simulink model "MazeRobot_start"  (R2018a)
settings: Solver=ode23t  StartTime=0.0  StopTime=inf  RelTol=1e-3
InitFcn:
  | RPInit
model workspace (MAT data in the model file):
  mapForSim.obsMap = [0 0 0 0 0 0 0 0 0 0 0 0 ... (40000 elements, 200x200)]
  mapForSim.scaleFactor = 25
  mapForSim.simMap = robotics.BinaryOccupancyGrid
  mapForSim.simMap.Grid = [1 1 1 1 1 1 1 1 1 1 1 1 ... (40000 elements, 200x200)]
  mapForSim.simMap.GridSize = [200 200]
  mapForSim.simMap.Resolution = 25
  occGrid = robotics.BinaryOccupancyGrid
  occGrid.Grid = [1 1 1 1 1 1 1 1 1 1 1 1 ... (40000 elements, 200x200)]
  occGrid.GridSize = [200 200]
  occGrid.Resolution = 25
undefined symbols (not defined in the file): X, Y, Z
libraries: sm_lib x19, RP_Simulator_Components x15, nesl_utility x11, RoboticsPlayground x5, Contact_Forces_Lib x2
settings Model: EnablePacing=on  Creator=josea  LastModifiedBy=josea
settings DebuggingCC: UnconnectedLineMsg=none
settings DiagnosticsConfigSet: SimMechanicsRigidlyBoundBlock=none
settings ExplorerConfigSet: InternalSimMechanicsExplorerSettings="<ExplorerConfiguration><canonicalview>default</canonicalview><AnimationSetting><BasePlaybackSpeed>1.0</BasePlaybackSpeed><PlaybackSpeedFactor>1.0</PlaybackSpeedFactor></AnimationSetting><TilePanel><TileInfo><Tiles Columns=\"1\" Count=\"1\" Rows=\"1\"><Column Weight=\"1\"/><Row Weight=\"1\"/><Tile Height=\"1\" Width=\"1\" X=\"0\" Y=\"0\"/></Tiles></TileInfo><SceneInfo><SceneViewer><BGColor><R>0.60000002384185791</R><G>0.60000002384185791</G><B>0.60000002384185791</B></BGColor><Camera><DoPerspective>off</DoPerspective><Position><X>2.71941451456511407</X><Y>-6.77816927707449679</Y><Z>7.37038703658607108</Z></Position><Center><X>-0.142764420925711066</X><Y>0.264709257438438761</Y><Z>0.243094267201064668</Z></Center><Up><X>-0.202833782227054393</X><Y>0.654576301685044992</Y><Z>0.728277640779805169</Z></Up><ViewLimDist>1</ViewLimDist><YLim>4.3228780116357628</YLim><XLim>5.31983664569920922</XLim></Camera></SceneViewer></SceneInfo></TilePanel><MechEditorPanel><Cameras/><GfxPanelCameraMap/><VideoCreator><PlaybackSpeedRatio>4.0</PlaybackSpeedRatio><FrameRate>30</FrameRate><VideoFormat>Motion JPEG AVI</VideoFormat><FrameSize>[1280 720]</FrameSize></VideoCreator></MechEditorPanel></ExplorerConfiguration>"

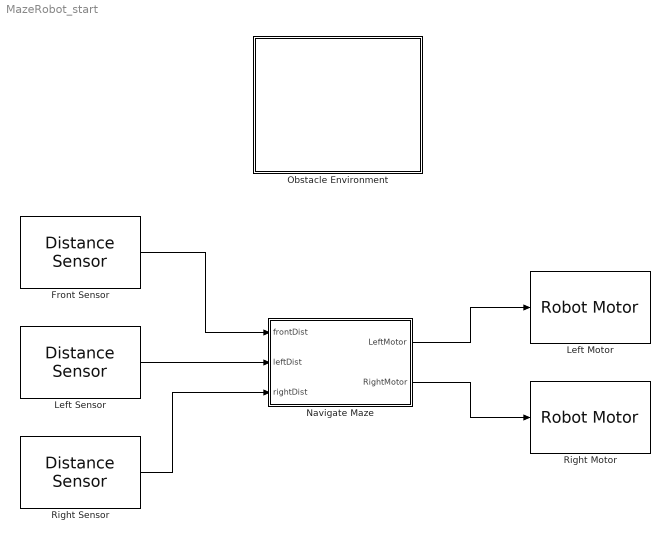
== system MazeRobot_start ==
  Front Sensor : RoboticsPlayground/Basic Sensors and Actuators/Distance Sensor  robotId=1  maxSenRange=10  minSenRange=0.02  senRes=0.01  sensOff=[0.25 0]  sensOffDeg=0  sensorTs=0.1
      settings: SourceProductName=Robotics Playground
  Left Motor : RoboticsPlayground/Basic Sensors and Actuators/Robot Motor  OverrideUsingVariant=Rbt1R  robotId=1  motorChoice=1
      settings: SourceProductName=Robotics Playground
  Left Sensor : RoboticsPlayground/Basic Sensors and Actuators/Distance Sensor  robotId=1  maxSenRange=10  minSenRange=0.02  senRes=0.01  sensOff=[0.15 0.15]  sensOffDeg=90  sensorTs=0.1
      settings: SourceProductName=Robotics Playground
  Navigate Maze : Stateflow chart  TreatAsAtomicUnit=on
  Obstacle Environment : Subsystem  mask(RP Obstacle Environment){obs1=on, obsPose1=[-2.042    0.091751], obsWidth1=3.713, obsLength1=0.91362, obs2=on, obsPose2=[0.025379    0.085895], obsWidth2=0.46852, obsLength2=4.6501, obs3=on, obsPose3=[1.3782      2.1357], obsWidth3=2.3075, obsLength3=0.57394, obs4=on, obsPose4=[1.2025     -1.9815], obsWidth4=2.776, obsLength4=0.51537, obs5=on, obsPose5=[2.8248   0.0097599], obsWidth5=2.1318, obsLength5=0.74963, obs6=on, obsPose6=[-2.1474      2.8736], obsWidth6=0.38653, obsLength6=1.9795, obs7=on, obsPose7=[-2.1415     -2.9244], obsWidth7=0.39824, obsLength7=1.9327, obs8=off, obsPose8=[2 2], obsWidth8=0.8, obsLength8=0.4, obs9=off, obsPose9=[2 2], obsWidth9=0.8, obsLength9=0.4, obs10=off, obsPose10=[2 2], obsWidth10=0.8, obsLength10=0.4, arenaLength=8, arenaWidth=8, robotId=1, wheelBase=0.5, wheelRadius=0.1, robotColor=[0 0 0.5], startPose=[-3.5 -3.5]}
      mask prompts: obs1 "Enable"; obsPose1 "Position X Y [m]"; obsWidth1 "Width [m]"; obsLength1 "Length [m]"; obs2 "Enable"; obsPose2 "Position X Y [m]"; obsWidth2 "Width [m]"; obsLength2 "Length [m]"; obs3 "Enable"; obsPose3 "Position X Y [m]"; obsWidth3 "Width [m]"; obsLength3 "Length [m]"; obs4 "Enable"; obsPose4 "Position X Y [m]"; obsWidth4 "Width [m]"; obsLength4 "Length [m]"; obs5 "Enable"; obsPose5 "Position X Y [m]"; obsWidth5 "Width [m]"; obsLength5 "Length [m]"; obs6 "Enable"; obsPose6 "Position X Y [m]"; obsWidth6 "Width [m]"; obsLength6 "Length [m]"; obs7 "Enable"; obsPose7 "Position X Y [m]"; obsWidth7 "Width [m]"; obsLength7 "Length [m]"; obs8 "Enable"; obsPose8 "Position X Y [m]"; obsWidth8 "Width [m]"; obsLength8 "Length [m]"; obs9 "Enable"; obsPose9 "Position X Y [m]"; obsWidth9 "Width [m]"; obsLength9 "Length [m]"; obs10 "Enable"; obsPose10 "Position X Y [m]"; obsWidth10 "Width [m]"; obsLength10 "Length [m]"; arenaLength "Length [m]"; arenaWidth "Width [m]"; robotId "Robot ID"; wheelBase "Distance between wheels [m]"; wheelRadius "Wheel radius [m]"; robotColor "Color [R G B]"; startPose "Initial Position X Y [m]"
      mask help:
      | This block contains a virtual environment for a single robot to interact with walls, obstacles and objects. Sensors implemented in the Robotics Playground library can be used to obtain environment information and actuators to interact with the robot behavior.
      |
      | Motor mapping for the robot is as follows:
      |
      | Motor 1 -> Left wheel motor torque
      | Motor 2 -> Right wheel motor torque
      settings: CopyFcn=|
      | set_param(gcs,'InitFcn','RPInit');
      | set_param(gcs,'Solver','ode23t');
      | set_param(gcs, 'EnablePacing', 'on')
      | set_param(gcs, 'PacingRate', 1)
      mask Help: web('obstacle_arena.htm')
      mask Callback obs1: commentObstacles(gcb)
      mask Callback obs2: commentObstacles(gcb)
      mask Callback obs3: commentObstacles(gcb)
      mask Callback obs4: commentObstacles(gcb)
      mask Callback obs5: commentObstacles(gcb)
      mask Callback obs6: commentObstacles(gcb)
      mask Callback obs7: commentObstacles(gcb)
      mask Callback obs8: commentObstacles(gcb)
      mask Callback obs9: commentObstacles(gcb)
      mask Callback obs10: commentObstacles(gcb)
      mask DialogControl obsT Prompt: Obstacle settings
      mask DialogControl Container19 Prompt: Set Obstacles Interactively
      mask DialogControl Control2 Prompt: Set Obstacles
      mask DialogControl Control2 Callback: setObstaclesUI(gcb)
      mask DialogControl Control3 Prompt: Disable all obstacles
      mask DialogControl Control3 Callback: disableObstacles(gcb)
      mask DialogControl Container21 Prompt: Obstacle Details
      mask DialogControl obsc1 Prompt: Obstacle 1
      mask DialogControl obsc2 Prompt: Obstacle 2
      mask DialogControl obsc3 Prompt: Obstacle 3
      mask DialogControl obsc4 Prompt: Obstacle 4
      mask DialogControl obsc5 Prompt: Obstacle 5
      mask DialogControl obsc6 Prompt: Obstacle 6
      mask DialogControl obsc7 Prompt: Obstacle 7
      mask DialogControl obsc8 Prompt: Obstacle 8
      mask DialogControl obsc9 Prompt: Obstacle 9
      mask DialogControl obsc10 Prompt: Obstacle 10
      mask DialogControl Container6 Prompt: Arena settings
      mask DialogControl Container4 Prompt: Robot settings
      mask Display:
      | color('white');
      | plot([100,100,100,100]*1,[100,100,100,100]*1);
      | plot([100,100,100,100]*0,[100,100,100,100]*0);
      | image('ObstacleEnv.PNG')
      | color('blue');
      | id=eval(get_param(gcb,'robotId'));
      | text(99, 92, ['Robot ID: ' num2str(id)], 'horizontalAlignment', 'right');
  Right Motor : RoboticsPlayground/Basic Sensors and Actuators/Robot Motor  OverrideUsingVariant=Rbt1R  robotId=1  motorChoice=2
      settings: SourceProductName=Robotics Playground
  Right Sensor : RoboticsPlayground/Basic Sensors and Actuators/Distance Sensor  robotId=1  maxSenRange=10  minSenRange=0.02  senRes=0.01  sensOff=[0.15 -0.15]  sensOffDeg=-90  sensorTs=0.1
      settings: SourceProductName=Robotics Playground
  wires:
  Navigate Maze/1(LeftMotor) -> Left Motor/1
  Navigate Maze/2(RightMotor) -> Right Motor/1
  Front Sensor/1 -> Navigate Maze/1(frontDist)
  Left Sensor/1 -> Navigate Maze/2(leftDist)
  Right Sensor/1 -> Navigate Maze/3(rightDist)

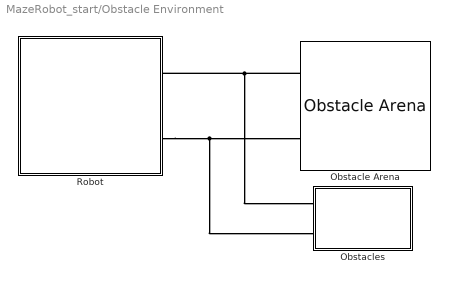
== system MazeRobot_start/Obstacle Environment ==
  Obstacle Arena : RP_Simulator_Components/Obstacle Arena  length=arenaLength  width=arenaWidth  robotRadius=wheelBase/2
  Obstacles : Subsystem
  Robot : Subsystem  AncestorBlock=RP_Simulator_Components/Contact Tank Robot  mask(RP Contact Tank Robot){robotId=robotId, wheelRadius=wheelRadius, wheelBase=wheelBase, wheelThickness=0.025, chassisThickness=0.05, startPose=startPose, choice=off, sensorTs=0.05, wheelMass=0.2, chassisMass=0.5, maxWheelTorque=1, floorSize=[arenaLength arenaWidth], wheelColor=[0.25 0.25 0.25], chassisColor=robotColor}
      mask prompts: robotId "Robot ID"; wheelRadius "Wheel Radius [m]"; wheelBase "Wheelbase [m]"; wheelThickness "Wheel Thickness [m]"; chassisThickness "Chassis Thickness [m]"; startPose "Start Position [m]"; choice "Reverse Start Position"; sensorTs "Sensor sample time [s]"; wheelMass "Wheel Mass [kg]"; chassisMass "Chassis Mass [kg]"; maxWheelTorque "Maximum wheel torque [N*m]"; floorSize "Floor Dimensions [m]"; wheelColor "Wheel Color"; chassisColor "Chassis Color"
      mask help:
      | This robot implements contact between the robot wheels and the floor of an arena. The stck-slip friction implemented using contact force libraries makes the robot behavior more realistic. The inputs to the robot are now motor torque, which is set using the Robotics Playground Motor blocks. The motor mappings are as follows:
      |
      | Motor 1 -> Left wheel motor torque
      | Motor 2 -> Right wheel motor torque
      mask init:
      | block=gcb;
      | ID=num2str(eval(get_param(block,'robotId')));
      | 
      | set_param([block '/motor1t'],'GotoTag',['R' ID 'motor1t']);
      | set_param([block '/motor2t'],'GotoTag',['R' ID 'motor2t']);
      | set_param([block '/motor1q'],'GotoTag',['R' ID 'motor1q']);
      | set_param([block '/motor1w'],'GotoTag',['R' ID 'motor1w']);
      | set_param([block '/motor2q'],'GotoTag',['R' ID 'motor2q']);
      | set_param([block '/motor2w'],'GotoTag',['R' ID 'motor2w']);
      | set_param([block '/xPose'],'GotoTag',['R' ID 'xPose']);
      | set_param([block '/yPose'],'GotoTag',['R' ID 'yPose']);
      | set_param([block '/tPose'],'GotoTag',['R' ID 'tPose']);
      | set_param([block '/tRate'],'GotoTag',['R' ID 'tRate']);
      | set_param([block '/tAngle'],'GotoTag',['R' ID 'tAngle']);
      | 
      | % Add sensor visuals
      | 
      | addSensors(block,eval(ID));
      mask DialogControl KinContainer Prompt: Kinematics
      mask DialogControl DynamicsContainer Prompt: Dynamics
      mask DialogControl AppearanceContainer Prompt: Appearance
      mask Display:
      | image('discRobot.PNG')
      | port_label('Rconn',1,'Robot')
      | port_label('Rconn',2,'Ref')
  connections:
  Obstacle Arena/LConn1 -- Obstacles/LConn1 -- Robot/RConn1
  Robot/RConn2 -- Obstacle Arena/LConn2 -- Obstacles/LConn2

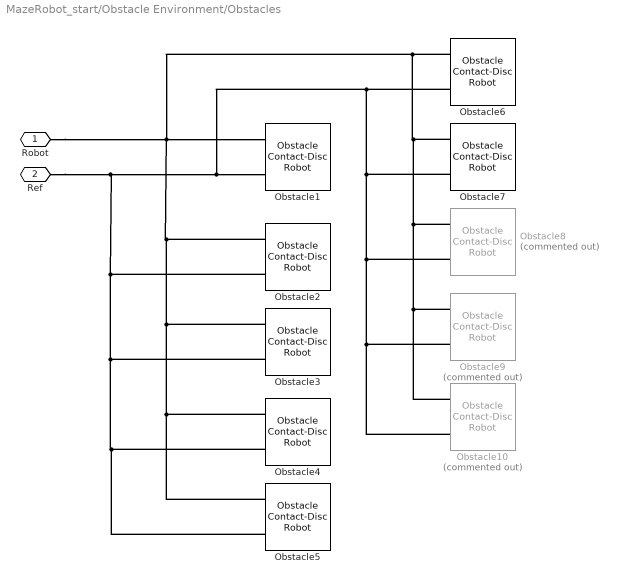
== system MazeRobot_start/Obstacle Environment/Obstacles ==
  Obstacle1 : RP_Simulator_Components/Obstacle Contact-Disc Robot  Pose=obsPose1  width=obsWidth1  length=obsLength1  robotRadius=wheelBase/2  height=0.3  color=[1.0 0.4 0.2]
      settings: SourceProductName=RP Simulator Components
  Obstacle10 : RP_Simulator_Components/Obstacle Contact-Disc Robot  Commented=on  Pose=obsPose10  width=obsWidth10  length=obsLength10  robotRadius=wheelBase/2  height=0.3  color=[1.0 0.4 0.2]
      settings: SourceProductName=RP Simulator Components
  Obstacle2 : RP_Simulator_Components/Obstacle Contact-Disc Robot  Pose=obsPose2  width=obsWidth2  length=obsLength2  robotRadius=wheelBase/2  height=0.3  color=[1.0 0.4 0.2]
      settings: SourceProductName=RP Simulator Components
  Obstacle3 : RP_Simulator_Components/Obstacle Contact-Disc Robot  Pose=obsPose3  width=obsWidth3  length=obsLength3  robotRadius=wheelBase/2  height=0.3  color=[1.0 0.4 0.2]
      settings: SourceProductName=RP Simulator Components
  Obstacle4 : RP_Simulator_Components/Obstacle Contact-Disc Robot  Pose=obsPose4  width=obsWidth4  length=obsLength4  robotRadius=wheelBase/2  height=0.3  color=[1.0 0.4 0.2]
      settings: SourceProductName=RP Simulator Components
  Obstacle5 : RP_Simulator_Components/Obstacle Contact-Disc Robot  Pose=obsPose5  width=obsWidth5  length=obsLength5  robotRadius=wheelBase/2  height=0.3  color=[1.0 0.4 0.2]
      settings: SourceProductName=RP Simulator Components
  Obstacle6 : RP_Simulator_Components/Obstacle Contact-Disc Robot  Pose=obsPose6  width=obsWidth6  length=obsLength6  robotRadius=wheelBase/2  height=0.3  color=[1.0 0.4 0.2]
      settings: SourceProductName=RP Simulator Components
  Obstacle7 : RP_Simulator_Components/Obstacle Contact-Disc Robot  Pose=obsPose7  width=obsWidth7  length=obsLength7  robotRadius=wheelBase/2  height=0.3  color=[1.0 0.4 0.2]
      settings: SourceProductName=RP Simulator Components
  Obstacle8 : RP_Simulator_Components/Obstacle Contact-Disc Robot  Commented=on  Pose=obsPose8  width=obsWidth8  length=obsLength8  robotRadius=wheelBase/2  height=0.3  color=[1.0 0.4 0.2]
      settings: SourceProductName=RP Simulator Components
  Obstacle9 : RP_Simulator_Components/Obstacle Contact-Disc Robot  Commented=on  Pose=obsPose9  width=obsWidth9  length=obsLength9  robotRadius=wheelBase/2  height=0.3  color=[1.0 0.4 0.2]
      settings: SourceProductName=RP Simulator Components
  Robot : PMIOPort  Side=Left
  Ref : PMIOPort  Port=2  Side=Left
  connections:
  Robot/RConn1 -- Obstacle10/LConn1 -- Obstacle9/LConn1 -- Obstacle8/LConn1 -- Obstacle7/LConn1 -- Obstacle6/LConn1 -- Obstacle5/LConn1 -- Obstacle4/LConn1 -- Obstacle3/LConn1 -- Obstacle2/LConn1 -- Obstacle1/LConn1
  Ref/RConn1 -- Obstacle5/LConn2 -- Obstacle4/LConn2 -- Obstacle3/LConn2 -- Obstacle2/LConn2 -- Obstacle7/LConn2 -- Obstacle8/LConn2 -- Obstacle9/LConn2 -- Obstacle10/LConn2 -- Obstacle6/LConn2 -- Obstacle1/LConn2

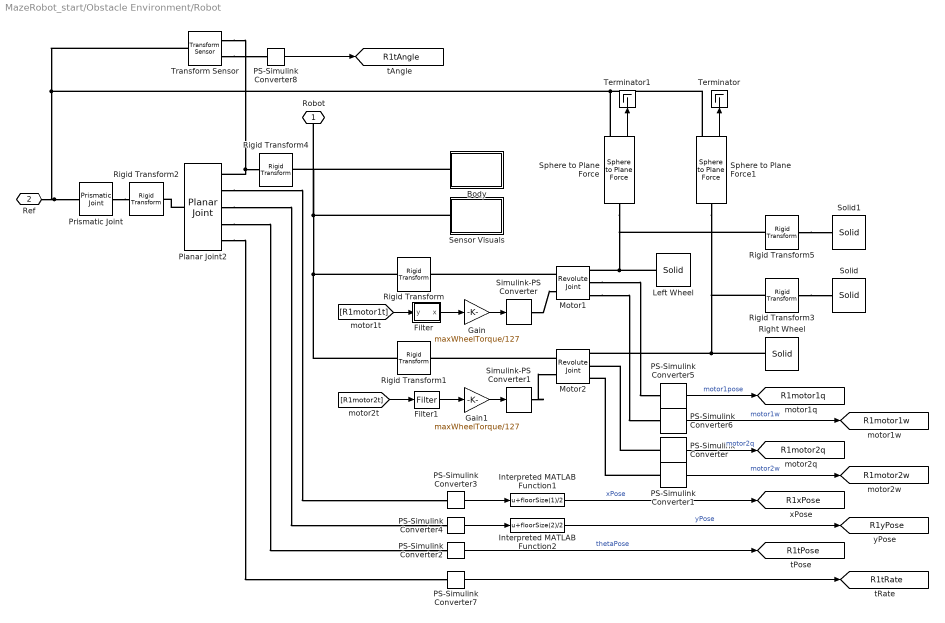
== system MazeRobot_start/Obstacle Environment/Robot ==
  Body : Subsystem
  Filter : Subsystem
  Filter1 : RP_Simulator_Components/Contact Tank Robot/Filter
      settings: SourceProductName=RP Simulator Components
  Gain : Gain  Gain=maxWheelTorque/127
  Gain1 : Gain  Gain=maxWheelTorque/127
  Interpreted MATLAB Function1 : MATLABFcn  MATLABFcn=u+floorSize(1)/2
  Interpreted MATLAB Function2 : MATLABFcn  MATLABFcn=u+floorSize(2)/2
  Left Wheel : sm_lib/Body Elements/Solid  InertiaType=CalculateFromGeometry  Mass=wheelMass  MassUnits=kg  CenterOfMass=[0 0 0]  CenterOfMassUnits=m  MomentsOfInertia=[1 1 1]  MomentsOfInertiaUnits=kg*m^2  ProductsOfInertia=[1 1 1]  ProductsOfInertiaUnits=kg*m^2  DensityBased=off  Density=1000  DensityUnits=kg/m^3  DoExposeReferenceFrame=on  SerializedFrames=<Frames/>  GraphicType=FromGeometry  MarkerShape=Sphere  MarkerSize=10  GraphicVisPropType=SimpleVisualProperties  GraphicDiffuseColor=wheelColor  GraphicSpecularColor=[0.5 0.5 0.5 1.0]  GraphicAmbientColor=[0.15 0.15 0.15 1.0]  GraphicEmissiveColor=[0.0 0.0 0.0 1.0]  GraphicShininess=75  GraphicOpacity=1.0  GeometryShape=Cylinder  RectangleSize=[1 1]  RectangleSizeUnits=m  BrickDimensions=[1 1 1]  BrickDimensionUnits=m  CylinderRadius=wheelRadius  CylinderRadiusUnits=m  CylinderLength=wheelThickness  CylinderLengthUnits=m  SphereRadius=1  SphereRadiusUnits=m  EllipsoidRadii=[1 1 1]  EllipsoidRadiiUnits=m  ExtrusionCrossSection=[1 1; -1 1; -1 -1; 1 -1]  ExtrusionCrossSectionUnits=m  ExtrusionLength=1  ExtrusionLengthUnits=m  PolygonNumSides=3  PolygonOuterRadius=1  PolygonOuterRadiusUnits=m  ExtGeomFileType=STEP  ExtGeomFileUnits=m  RevolutionCrossSection=[1 1; 1 -1; 2 -1; 2 1]  RevolutionCrossSectionUnits=m  RevolutionExtent=Full  RevolutionAngle=180  RevolutionAngleUnits=deg
  Motor1 : sm_lib/Joints/Revolute Joint  SenseConstraintForce=off  SenseConstraintForceX=off  SenseConstraintForceY=off  SenseConstraintForceZ=off  SenseConstraintTorque=off  SenseConstraintTorqueX=off  SenseConstraintTorqueY=off  SenseConstraintTorqueZ=off  SenseTotalForce=off  SenseTotalForceX=off  SenseTotalForceY=off  SenseTotalForceZ=off  SenseTotalTorque=off  SenseTotalTorqueX=off  SenseTotalTorqueY=off  SenseTotalTorqueZ=off  CompositeWrenchDir=FollowerOnBase  CompositeWrenchFrame=BaseFrame  EquilibriumPosition=0  EquilibriumPositionUnits=deg  SpringStiffness=0  SpringStiffnessUnits=N*m/deg  DampingCoefficient=0.004  DampingCoefficientUnits=N*m/(deg/s)  TorqueActuationMode=InputTorque  MotionActuationMode=ComputedMotion  SensePosition=on  SenseVelocity=on  SenseAcceleration=off  SenseTorqueForce=off  PositionTargetSpecify=off  PositionTargetPriority=High  PositionTargetValue=0  PositionTargetValueUnits=deg  VelocityTargetSpecify=off  VelocityTargetPriority=High  VelocityTargetValue=0  VelocityTargetValueUnits=deg/s
  Motor2 : sm_lib/Joints/Revolute Joint  SenseConstraintForce=off  SenseConstraintForceX=off  SenseConstraintForceY=off  SenseConstraintForceZ=off  SenseConstraintTorque=off  SenseConstraintTorqueX=off  SenseConstraintTorqueY=off  SenseConstraintTorqueZ=off  SenseTotalForce=off  SenseTotalForceX=off  SenseTotalForceY=off  SenseTotalForceZ=off  SenseTotalTorque=off  SenseTotalTorqueX=off  SenseTotalTorqueY=off  SenseTotalTorqueZ=off  CompositeWrenchDir=FollowerOnBase  CompositeWrenchFrame=BaseFrame  EquilibriumPosition=0  EquilibriumPositionUnits=deg  SpringStiffness=0  SpringStiffnessUnits=N*m/deg  DampingCoefficient=0.004  DampingCoefficientUnits=N*m/(deg/s)  TorqueActuationMode=InputTorque  MotionActuationMode=ComputedMotion  SensePosition=on  SenseVelocity=on  SenseAcceleration=off  SenseTorqueForce=off  PositionTargetSpecify=off  PositionTargetPriority=High  PositionTargetValue=0  PositionTargetValueUnits=deg  VelocityTargetSpecify=off  VelocityTargetPriority=High  VelocityTargetValue=0  VelocityTargetValueUnits=deg/s
  PS-Simulink Converter{,1,3..6} (6 alike) : nesl_utility/PS-Simulink Converter  PhysicalDomain=network_engine_domain  SubClassName=ps_output  LeftPortType=input  RightPortType=output  PseudoPeriodic=off  Frequencies=[]  Unit=1  AffineConversion=off
  PS-Simulink Converter2 : nesl_utility/PS-Simulink Converter  PhysicalDomain=network_engine_domain  SubClassName=ps_output  LeftPortType=input  RightPortType=output  PseudoPeriodic=off  Frequencies=[]  Unit=rad  AffineConversion=off
  PS-Simulink Converter7 : nesl_utility/PS-Simulink Converter  PhysicalDomain=network_engine_domain  SubClassName=ps_output  LeftPortType=input  RightPortType=output  PseudoPeriodic=off  Frequencies=[]  Unit=deg/s  AffineConversion=off
  PS-Simulink Converter8 : nesl_utility/PS-Simulink Converter  PhysicalDomain=network_engine_domain  SubClassName=ps_output  LeftPortType=input  RightPortType=output  PseudoPeriodic=off  Frequencies=[]  Unit=deg  AffineConversion=off
  Planar Joint2 : sm_lib/Joints/Planar Joint  SenseConstraintForce=off  SenseConstraintForceX=off  SenseConstraintForceY=off  SenseConstraintForceZ=off  SenseConstraintTorque=off  SenseConstraintTorqueX=off  SenseConstraintTorqueY=off  SenseConstraintTorqueZ=off  SenseTotalForce=off  SenseTotalForceX=off  SenseTotalForceY=off  SenseTotalForceZ=off  SenseTotalTorque=off  SenseTotalTorqueX=off  SenseTotalTorqueY=off  SenseTotalTorqueZ=off  CompositeWrenchDir=FollowerOnBase  CompositeWrenchFrame=BaseFrame  PxEquilibriumPosition=0  PxEquilibriumPositionUnits=m  PxSpringStiffness=0  PxSpringStiffnessUnits=N/m  PxDampingCoefficient=5  PxDampingCoefficientUnits=N/(m/s)  PxTorqueActuationMode=NoTorque  PxMotionActuationMode=ComputedMotion  PxSensePosition=on  PxSenseVelocity=off  PxSenseAcceleration=off  PxSenseTorqueForce=off  PxPositionTargetSpecify=on  PxPositionTargetPriority=High  PxPositionTargetValue=startPose(1)  PxPositionTargetValueUnits=m  PxVelocityTargetSpecify=off  PxVelocityTargetPriority=High  PxVelocityTargetValue=0  PxVelocityTargetValueUnits=m/s  PyEquilibriumPosition=0  PyEquilibriumPositionUnits=m  PySpringStiffness=0  PySpringStiffnessUnits=N/m  PyDampingCoefficient=5  PyDampingCoefficientUnits=N/(m/s)  PyTorqueActuationMode=NoTorque  PyMotionActuationMode=ComputedMotion  PySensePosition=on  PySenseVelocity=off  PySenseAcceleration=off  PySenseTorqueForce=off  PyPositionTargetSpecify=on  PyPositionTargetPriority=High  PyPositionTargetValue=startPose(2)  PyPositionTargetValueUnits=m  PyVelocityTargetSpecify=off  PyVelocityTargetPriority=High  PyVelocityTargetValue=0  PyVelocityTargetValueUnits=m/s  RzEquilibriumPosition=0  RzEquilibriumPositionUnits=deg  RzSpringStiffness=0  RzSpringStiffnessUnits=N*m/deg  RzDampingCoefficient=2/45  RzDampingCoefficientUnits=N*m/(deg/s)  RzTorqueActuationMode=NoTorque  RzMotionActuationMode=ComputedMotion  RzSensePosition=on  RzSenseVelocity=on  RzSenseAcceleration=off  RzSenseTorqueForce=off  RzPositionTargetSpecify=off  RzPositionTargetPriority=High  RzPositionTargetValue=0  RzPositionTargetValueUnits=deg  RzVelocityTargetSpecify=off  RzVelocityTargetPriority=High  RzVelocityTargetValue=0  RzVelocityTargetValueUnits=deg/s
  Prismatic Joint : sm_lib/Joints/Prismatic Joint  SenseConstraintForce=off  SenseConstraintForceX=off  SenseConstraintForceY=off  SenseConstraintForceZ=off  SenseConstraintTorque=off  SenseConstraintTorqueX=off  SenseConstraintTorqueY=off  SenseConstraintTorqueZ=off  SenseTotalForce=off  SenseTotalForceX=off  SenseTotalForceY=off  SenseTotalForceZ=off  SenseTotalTorque=off  SenseTotalTorqueX=off  SenseTotalTorqueY=off  SenseTotalTorqueZ=off  CompositeWrenchDir=FollowerOnBase  CompositeWrenchFrame=BaseFrame  EquilibriumPosition=0  EquilibriumPositionUnits=m  SpringStiffness=0  SpringStiffnessUnits=N/m  DampingCoefficient=0  DampingCoefficientUnits=N/(m/s)  TorqueActuationMode=NoTorque  MotionActuationMode=ComputedMotion  SensePosition=off  SenseVelocity=off  SenseAcceleration=off  SenseTorqueForce=off  PositionTargetSpecify=on  PositionTargetPriority=High  PositionTargetValue=0.02  PositionTargetValueUnits=m  VelocityTargetSpecify=off  VelocityTargetPriority=High  VelocityTargetValue=0  VelocityTargetValueUnits=m/s
  Right Wheel : sm_lib/Body Elements/Solid  InertiaType=CalculateFromGeometry  Mass=wheelMass  MassUnits=kg  CenterOfMass=[0 0 0]  CenterOfMassUnits=m  MomentsOfInertia=[1 1 1]  MomentsOfInertiaUnits=kg*m^2  ProductsOfInertia=[1 1 1]  ProductsOfInertiaUnits=kg*m^2  DensityBased=off  Density=1000  DensityUnits=kg/m^3  DoExposeReferenceFrame=on  SerializedFrames=<Frames/>  GraphicType=FromGeometry  MarkerShape=Sphere  MarkerSize=10  GraphicVisPropType=SimpleVisualProperties  GraphicDiffuseColor=wheelColor  GraphicSpecularColor=[0.5 0.5 0.5 1.0]  GraphicAmbientColor=[0.15 0.15 0.15 1.0]  GraphicEmissiveColor=[0.0 0.0 0.0 1.0]  GraphicShininess=75  GraphicOpacity=1.0  GeometryShape=Cylinder  RectangleSize=[1 1]  RectangleSizeUnits=m  BrickDimensions=[1 1 1]  BrickDimensionUnits=m  CylinderRadius=wheelRadius  CylinderRadiusUnits=m  CylinderLength=wheelThickness  CylinderLengthUnits=m  SphereRadius=1  SphereRadiusUnits=m  EllipsoidRadii=[1 1 1]  EllipsoidRadiiUnits=m  ExtrusionCrossSection=[1 1; -1 1; -1 -1; 1 -1]  ExtrusionCrossSectionUnits=m  ExtrusionLength=1  ExtrusionLengthUnits=m  PolygonNumSides=3  PolygonOuterRadius=1  PolygonOuterRadiusUnits=m  ExtGeomFileType=STEP  ExtGeomFileUnits=m  RevolutionCrossSection=[1 1; 1 -1; 2 -1; 2 1]  RevolutionCrossSectionUnits=m  RevolutionExtent=Full  RevolutionAngle=180  RevolutionAngleUnits=deg
  Rigid Transform : sm_lib/Frames and Transforms/Rigid Transform  TranslationMethod=StandardAxis  TranslationStandardOffset=wheelBase/2  TranslationLengthUnit=m  TranslationStandardAxis=+Y  TranslationCartesianOffset=[0 0 0]  TranslationROffset=0  TranslationROffsetUnits=m  TranslationZOffset=0  TranslationZOffsetUnits=m  TranslationThetaOffset=0  TranslationThetaOffsetUnits=deg  RotationMethod=AlignedAxes  RotationAngleUnits=deg  RotationStandardAxis=+Z  RotationAngle=0.0  RotationArbitraryAxis=[0 0 1]  FollAlignAxisA=+Z  BaseAlignAxisA=+Y  FollAlignAxisB=+X  BaseAlignAxisB=+X  RotationSequenceAxes=FollowerAxes  RotationSequence=XYX  RotationSequenceAngles=[0 0 0]  RotationSequenceAnglesUnits=deg  RotationMatrix=[1 0 0; 0 1 0; 0 0 1]
  Rigid Transform1 : sm_lib/Frames and Transforms/Rigid Transform  TranslationMethod=StandardAxis  TranslationStandardOffset=wheelBase/2  TranslationLengthUnit=m  TranslationStandardAxis=-Y  TranslationCartesianOffset=[0 0 0]  TranslationROffset=0  TranslationROffsetUnits=m  TranslationZOffset=0  TranslationZOffsetUnits=m  TranslationThetaOffset=0  TranslationThetaOffsetUnits=deg  RotationMethod=AlignedAxes  RotationAngleUnits=deg  RotationStandardAxis=+Z  RotationAngle=0.0  RotationArbitraryAxis=[0 0 1]  FollAlignAxisA=+Z  BaseAlignAxisA=+Y  FollAlignAxisB=+X  BaseAlignAxisB=+X  RotationSequenceAxes=FollowerAxes  RotationSequence=XYX  RotationSequenceAngles=[0 0 0]  RotationSequenceAnglesUnits=deg  RotationMatrix=[1 0 0; 0 1 0; 0 0 1]
  Rigid Transform2 : sm_lib/Frames and Transforms/Rigid Transform  TranslationMethod=StandardAxis  TranslationStandardOffset=wheelRadius  TranslationLengthUnit=m  TranslationStandardAxis=+Z  TranslationCartesianOffset=[0 0 0]  TranslationROffset=0  TranslationROffsetUnits=m  TranslationZOffset=0  TranslationZOffsetUnits=m  TranslationThetaOffset=0  TranslationThetaOffsetUnits=deg  RotationMethod=None  RotationAngleUnits=deg  RotationStandardAxis=+Z  RotationAngle=0.0  RotationArbitraryAxis=[0 0 1]  FollAlignAxisA=+Z  BaseAlignAxisA=+Y  FollAlignAxisB=+X  BaseAlignAxisB=+X  RotationSequenceAxes=FollowerAxes  RotationSequence=XYX  RotationSequenceAngles=[0 0 0]  RotationSequenceAnglesUnits=deg  RotationMatrix=[1 0 0; 0 1 0; 0 0 1]
  Rigid Transform3 : sm_lib/Frames and Transforms/Rigid Transform  TranslationMethod=Cartesian  TranslationStandardOffset=0  TranslationLengthUnit=m  TranslationStandardAxis=+Z  TranslationCartesianOffset=[wheelRadius/2 0 0]  TranslationROffset=0  TranslationROffsetUnits=m  TranslationZOffset=0  TranslationZOffsetUnits=m  TranslationThetaOffset=0  TranslationThetaOffsetUnits=deg  RotationMethod=None  RotationAngleUnits=deg  RotationStandardAxis=+Z  RotationAngle=0.0  RotationArbitraryAxis=[0 0 1]  FollAlignAxisA=+X  BaseAlignAxisA=+Y  FollAlignAxisB=+Y  BaseAlignAxisB=+Z  RotationSequenceAxes=FollowerAxes  RotationSequence=XYX  RotationSequenceAngles=[0 0 0]  RotationSequenceAnglesUnits=deg  RotationMatrix=[1 0 0; 0 1 0; 0 0 1]
  Rigid Transform4 : sm_lib/Frames and Transforms/Rigid Transform  TranslationMethod=None  TranslationStandardOffset=0  TranslationLengthUnit=m  TranslationStandardAxis=+Z  TranslationCartesianOffset=[0 0 0]  TranslationROffset=0  TranslationROffsetUnits=m  TranslationZOffset=0  TranslationZOffsetUnits=m  TranslationThetaOffset=0  TranslationThetaOffsetUnits=deg  RotationMethod=StandardAxis  RotationAngleUnits=deg  RotationStandardAxis=+Z  RotationAngle=180*choice  RotationArbitraryAxis=[0 0 1]  FollAlignAxisA=+X  BaseAlignAxisA=+Y  FollAlignAxisB=+Y  BaseAlignAxisB=+Z  RotationSequenceAxes=FollowerAxes  RotationSequence=XYX  RotationSequenceAngles=[0 0 0]  RotationSequenceAnglesUnits=deg  RotationMatrix=[1 0 0; 0 1 0; 0 0 1]
  Rigid Transform5 : sm_lib/Frames and Transforms/Rigid Transform  TranslationMethod=Cartesian  TranslationStandardOffset=0  TranslationLengthUnit=m  TranslationStandardAxis=+Z  TranslationCartesianOffset=[wheelRadius/2 0 0]  TranslationROffset=0  TranslationROffsetUnits=m  TranslationZOffset=0  TranslationZOffsetUnits=m  TranslationThetaOffset=0  TranslationThetaOffsetUnits=deg  RotationMethod=None  RotationAngleUnits=deg  RotationStandardAxis=+Z  RotationAngle=0.0  RotationArbitraryAxis=[0 0 1]  FollAlignAxisA=+X  BaseAlignAxisA=+Y  FollAlignAxisB=+Y  BaseAlignAxisB=+Z  RotationSequenceAxes=FollowerAxes  RotationSequence=XYX  RotationSequenceAngles=[0 0 0]  RotationSequenceAnglesUnits=deg  RotationMatrix=[1 0 0; 0 1 0; 0 0 1]
  Sensor Visuals : Subsystem
  Simulink-PS Converter : nesl_utility/Simulink-PS Converter  PhysicalDomain=network_engine_domain  SubClassName=ps_input  LeftPortType=input  RightPortType=output  PseudoPeriodic=off  Frequencies=[]  NoiseDistribution=none  NoiseParameters=[]  Unit=1  AffineConversion=off  FilteringAndDerivatives=provide  SimscapeFilterOrder=1  InputFilterTimeConstant=0.05  UdotUserProvided=0
  Simulink-PS Converter1 : nesl_utility/Simulink-PS Converter  PhysicalDomain=network_engine_domain  SubClassName=ps_input  LeftPortType=input  RightPortType=output  PseudoPeriodic=off  Frequencies=[]  NoiseDistribution=none  NoiseParameters=[]  Unit=1  AffineConversion=off  FilteringAndDerivatives=provide  SimscapeFilterOrder=1  InputFilterTimeConstant=0.05  UdotUserProvided=0
  Solid : sm_lib/Body Elements/Solid  InertiaType=CalculateFromGeometry  Mass=1  MassUnits=kg  CenterOfMass=[0 0 0]  CenterOfMassUnits=m  MomentsOfInertia=[1 1 1]  MomentsOfInertiaUnits=kg*m^2  ProductsOfInertia=[1 1 1]  ProductsOfInertiaUnits=kg*m^2  DensityBased=on  Density=1000  DensityUnits=kg/m^3  DoExposeReferenceFrame=on  SerializedFrames=<Frames/>  GraphicType=FromGeometry  MarkerShape=Sphere  MarkerSize=10  GraphicVisPropType=SimpleVisualProperties  GraphicDiffuseColor=[0.0 0.8 0.8]  GraphicSpecularColor=[0.5 0.5 0.5 1.0]  GraphicAmbientColor=[0.15 0.15 0.15 1.0]  GraphicEmissiveColor=[0.0 0.0 0.0 1.0]  GraphicShininess=75  GraphicOpacity=1.0  GeometryShape=Brick  RectangleSize=[1 1]  RectangleSizeUnits=m  BrickDimensions=[wheelRadius*0.8 wheelThickness*1.05 wheelThickness*1.05]  BrickDimensionUnits=m  CylinderRadius=1  CylinderRadiusUnits=m  CylinderLength=1  CylinderLengthUnits=m  SphereRadius=1  SphereRadiusUnits=m  EllipsoidRadii=[1 1 1]  EllipsoidRadiiUnits=m  ExtrusionCrossSection=[1 1; -1 1; -1 -1; 1 -1]  ExtrusionCrossSectionUnits=m  ExtrusionLength=1  ExtrusionLengthUnits=m  PolygonNumSides=3  PolygonOuterRadius=1  PolygonOuterRadiusUnits=m  ExtGeomFileType=STEP  ExtGeomFileUnits=m  RevolutionCrossSection=[1 1; 1 -1; 2 -1; 2 1]  RevolutionCrossSectionUnits=m  RevolutionExtent=Full  RevolutionAngle=180  RevolutionAngleUnits=deg
  Solid1 : sm_lib/Body Elements/Solid  InertiaType=CalculateFromGeometry  Mass=1  MassUnits=kg  CenterOfMass=[0 0 0]  CenterOfMassUnits=m  MomentsOfInertia=[1 1 1]  MomentsOfInertiaUnits=kg*m^2  ProductsOfInertia=[1 1 1]  ProductsOfInertiaUnits=kg*m^2  DensityBased=on  Density=1000  DensityUnits=kg/m^3  DoExposeReferenceFrame=on  SerializedFrames=<Frames/>  GraphicType=FromGeometry  MarkerShape=Sphere  MarkerSize=10  GraphicVisPropType=SimpleVisualProperties  GraphicDiffuseColor=[0.0 0.8 0.8]  GraphicSpecularColor=[0.5 0.5 0.5 1.0]  GraphicAmbientColor=[0.15 0.15 0.15 1.0]  GraphicEmissiveColor=[0.0 0.0 0.0 1.0]  GraphicShininess=75  GraphicOpacity=1.0  GeometryShape=Brick  RectangleSize=[1 1]  RectangleSizeUnits=m  BrickDimensions=[wheelRadius*0.8 wheelThickness*1.05 wheelThickness*1.05]  BrickDimensionUnits=m  CylinderRadius=1  CylinderRadiusUnits=m  CylinderLength=1  CylinderLengthUnits=m  SphereRadius=1  SphereRadiusUnits=m  EllipsoidRadii=[1 1 1]  EllipsoidRadiiUnits=m  ExtrusionCrossSection=[1 1; -1 1; -1 -1; 1 -1]  ExtrusionCrossSectionUnits=m  ExtrusionLength=1  ExtrusionLengthUnits=m  PolygonNumSides=3  PolygonOuterRadius=1  PolygonOuterRadiusUnits=m  ExtGeomFileType=STEP  ExtGeomFileUnits=m  RevolutionCrossSection=[1 1; 1 -1; 2 -1; 2 1]  RevolutionCrossSectionUnits=m  RevolutionExtent=Full  RevolutionAngle=180  RevolutionAngleUnits=deg
  Sphere to Plane Force : Contact_Forces_Lib/3D/Sphere to Plane Force  sphere_rad=wheelRadius  plane_lenx=floorSize(1)  plane_leny=floorSize(2)  plane_depth=0.01/2  force_law=Linear  k_contact=1e4  b_contact=1e2  pen_full_damp_F=1e-4  pen_exponent=1  custom_param_1=1  custom_param_2=1  friction_law=Stick-Slip Continuous  mu_kinetic=0.5  mu_static=0.7  v_thr=0.001  vis_on=off  vis_opc_en=0  vis_len_plaBz=0.005  vis_clr=[0.9 0.2 0.2]  vis_opc=0.7
  Sphere to Plane Force1 : Contact_Forces_Lib/3D/Sphere to Plane Force  sphere_rad=wheelRadius  plane_lenx=floorSize(1)  plane_leny=floorSize(2)  plane_depth=0.01/2  force_law=Linear  k_contact=1e4  b_contact=1e2  pen_full_damp_F=1e-4  pen_exponent=1  custom_param_1=1  custom_param_2=1  friction_law=Stick-Slip Continuous  mu_kinetic=0.5  mu_static=0.7  v_thr=0.001  vis_on=off  vis_opc_en=0  vis_len_plaBz=0.005  vis_clr=[0.9 0.2 0.2]  vis_opc=0.7
  Terminator : Terminator
  Terminator1 : Terminator
  Transform Sensor : sm_lib/Frames and Transforms/Transform Sensor  MeasurementFrame=World  SenseAngle=on  SenseAxis=off  SenseAngle1=off  SenseAngle2=off  SenseAngle3=off  SenseQ=off  SenseR=off  SenseOmegaX=off  SenseOmegaY=off  SenseOmegaZ=off  SenseOmega1=off  SenseOmega2=off  SenseOmega3=off  SenseQDot=off  SenseRDot=off  SenseAlphaX=off  SenseAlphaY=off  SenseAlphaZ=off  SenseAlpha1=off  SenseAlpha2=off  SenseAlpha3=off  SenseQDDot=off  SenseRDDot=off  SenseX=off  SenseY=off  SenseZ=off  SenseRad=off  SenseAzim=off  SenseDist=off  SenseInc=off  SenseXDot=off  SenseYDot=off  SenseZDot=off  SenseRadDot=off  SenseAzimDot=off  SenseDistDot=off  SenseIncDot=off  SenseXDDot=off  SenseYDDot=off  SenseZDDot=off  SenseRadDDot=off  SenseAzimDDot=off  SenseDistDDot=off  SenseIncDDot=off
  Robot : PMIOPort  Side=Right
  Ref : PMIOPort  Port=2  Side=Right
  tag scope: R1motor1q=global, R1motor1w=global, R1motor2q=global, R1motor2w=global, R1tAngle=global, R1tPose=global, R1tRate=global, R1xPose=global, R1yPose=global
  wires:
  [R1motor2t] -> Filter1/1
  [R1motor1t] -> Filter/1(y)
  Gain1/1 -> Simulink-PS Converter1/1
  Gain/1 -> Simulink-PS Converter/1
  Filter/1(x) -> Gain/1
  Filter1/1 -> Gain1/1
  Sphere to Plane Force1/1 -> Terminator/1
  Sphere to Plane Force/1 -> Terminator1/1
  PS-Simulink Converter4/1 -> Interpreted MATLAB Function2/1
  PS-Simulink Converter3/1 -> Interpreted MATLAB Function1/1
  PS-Simulink Converter2/1 -> [R1tPose]  "thetaPose"
  Interpreted MATLAB Function1/1 -> [R1xPose]  "xPose"
  Interpreted MATLAB Function2/1 -> [R1yPose]  "yPose"
  PS-Simulink Converter1/1 -> [R1motor2w]  "motor2w"
  PS-Simulink Converter/1 -> [R1motor2q]  "motor2q"
  PS-Simulink Converter5/1 -> [R1motor1q]  "motor1pose"
  PS-Simulink Converter6/1 -> [R1motor1w]  "motor1w"
  PS-Simulink Converter7/1 -> [R1tRate]
  PS-Simulink Converter8/1 -> [R1tAngle]
  connections:
  Prismatic Joint/RConn1 -- Rigid Transform2/LConn1
  Transform Sensor/RConn1 -- Rigid Transform4/LConn1 -- Planar Joint2/RConn1
  Rigid Transform1/LConn1 -- Sensor Visuals/LConn1 -- Robot/RConn1 -- Body/LConn1 -- Rigid Transform4/RConn1 -- Rigid Transform/LConn1
  Left Wheel/RConn1 -- Motor1/RConn1 -- Rigid Transform5/LConn1 -- Sphere to Plane Force/LConn1
  Motor2/LConn1 -- Rigid Transform1/RConn1
  Sphere to Plane Force1/RConn1 -- Sphere to Plane Force/RConn1 -- Prismatic Joint/LConn1 -- Ref/RConn1 -- Transform Sensor/LConn1
  Planar Joint2/LConn1 -- Rigid Transform2/RConn1
  Motor1/LConn1 -- Rigid Transform/RConn1
  Right Wheel/RConn1 -- Motor2/RConn1 -- Rigid Transform3/LConn1 -- Sphere to Plane Force1/LConn1
  Simulink-PS Converter1/RConn1 -- Motor2/LConn2
  Simulink-PS Converter/RConn1 -- Motor1/LConn2
  Planar Joint2/RConn2 -- PS-Simulink Converter3/LConn1
  Planar Joint2/RConn3 -- PS-Simulink Converter4/LConn1
  Planar Joint2/RConn4 -- PS-Simulink Converter2/LConn1
  Motor1/RConn2 -- PS-Simulink Converter5/LConn1
  Motor1/RConn3 -- PS-Simulink Converter6/LConn1
  PS-Simulink Converter/LConn1 -- Motor2/RConn2
  PS-Simulink Converter1/LConn1 -- Motor2/RConn3
  Rigid Transform3/RConn1 -- Solid/RConn1
  Rigid Transform5/RConn1 -- Solid1/RConn1
  Planar Joint2/RConn5 -- PS-Simulink Converter7/LConn1
  Transform Sensor/RConn2 -- PS-Simulink Converter8/LConn1

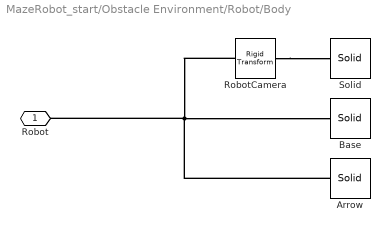
== system MazeRobot_start/Obstacle Environment/Robot/Body ==
  Arrow : sm_lib/Body Elements/Solid  InertiaType=PointMass  Mass=0.2  MassUnits=kg  CenterOfMass=[0 0 0]  CenterOfMassUnits=m  MomentsOfInertia=[1 1 1]  MomentsOfInertiaUnits=kg*m^2  ProductsOfInertia=[1 1 1]  ProductsOfInertiaUnits=kg*m^2  DensityBased=on  Density=1000  DensityUnits=kg/m^3  DoExposeReferenceFrame=on  SerializedFrames=<Frames/>  GraphicType=FromGeometry  MarkerShape=Sphere  MarkerSize=10  GraphicVisPropType=SimpleVisualProperties  GraphicDiffuseColor=[0.8 0.0 1.0]  GraphicSpecularColor=[0.5 0.5 0.5 1.0]  GraphicAmbientColor=[0.15 0.15 0.15 1.0]  GraphicEmissiveColor=[0.0 0.0 0.0 1.0]  GraphicShininess=75  GraphicOpacity=1.0  GeometryShape=RegularExtrusion  RectangleSize=[1 1]  RectangleSizeUnits=m  BrickDimensions=[1 1 1]  BrickDimensionUnits=m  CylinderRadius=1  CylinderRadiusUnits=m  CylinderLength=1  CylinderLengthUnits=m  SphereRadius=1  SphereRadiusUnits=m  EllipsoidRadii=[1 1 1]  EllipsoidRadiiUnits=m  ExtrusionCrossSection=[1 1; -1 1; -1 -1; 1 -1]  ExtrusionCrossSectionUnits=m  ExtrusionLength=1.3*chassisThickness  ExtrusionLengthUnits=m  PolygonNumSides=3  PolygonOuterRadius=wheelBase/2-wheelBase*0.15  PolygonOuterRadiusUnits=m  ExtGeomFileType=STEP  ExtGeomFileUnits=m  RevolutionCrossSection=[0 0.15; 0 -0.15; 0.15 -0.15]  RevolutionCrossSectionUnits=m  RevolutionExtent=Full  RevolutionAngle=180  RevolutionAngleUnits=deg
  Base : sm_lib/Body Elements/Solid  InertiaType=CalculateFromGeometry  Mass=chassisMass  MassUnits=kg  CenterOfMass=[0 0 0]  CenterOfMassUnits=m  MomentsOfInertia=[1 1 1]  MomentsOfInertiaUnits=kg*m^2  ProductsOfInertia=[1 1 1]  ProductsOfInertiaUnits=kg*m^2  DensityBased=off  Density=chassisMass  DensityUnits=kg/m^3  DoExposeReferenceFrame=on  SerializedFrames=<Frames/>  GraphicType=FromGeometry  MarkerShape=Sphere  MarkerSize=10  GraphicVisPropType=SimpleVisualProperties  GraphicDiffuseColor=chassisColor  GraphicSpecularColor=[0.5 0.5 0.5 1.0]  GraphicAmbientColor=[0.15 0.15 0.15 1.0]  GraphicEmissiveColor=[0.0 0.0 0.0 1.0]  GraphicShininess=75  GraphicOpacity=1.0  GeometryShape=Cylinder  RectangleSize=[1 1]  RectangleSizeUnits=m  BrickDimensions=[1 1 1]  BrickDimensionUnits=m  CylinderRadius=(wheelBase-wheelThickness)/2  CylinderRadiusUnits=m  CylinderLength=chassisThickness  CylinderLengthUnits=m  SphereRadius=1  SphereRadiusUnits=m  EllipsoidRadii=[1 1 1]  EllipsoidRadiiUnits=m  ExtrusionCrossSection=[1 1; -1 1; -1 -1; 1 -1]  ExtrusionCrossSectionUnits=m  ExtrusionLength=1  ExtrusionLengthUnits=m  PolygonNumSides=3  PolygonOuterRadius=1  PolygonOuterRadiusUnits=m  ExtGeomFileType=STEP  ExtGeomFileUnits=m  RevolutionCrossSection=[1 1; 1 -1; 2 -1; 2 1]  RevolutionCrossSectionUnits=m  RevolutionExtent=Full  RevolutionAngle=180  RevolutionAngleUnits=deg
  RobotCamera : sm_lib/Frames and Transforms/Rigid Transform  TranslationMethod=Cartesian  TranslationStandardOffset=0  TranslationLengthUnit=m  TranslationStandardAxis=+Z  TranslationCartesianOffset=[-0.5 0 0.35]  TranslationROffset=0  TranslationROffsetUnits=m  TranslationZOffset=0  TranslationZOffsetUnits=m  TranslationThetaOffset=0  TranslationThetaOffsetUnits=deg  RotationMethod=StandardAxis  RotationAngleUnits=deg  RotationStandardAxis=+Y  RotationAngle=20  RotationArbitraryAxis=[0 0 1]  FollAlignAxisA=+X  BaseAlignAxisA=+Y  FollAlignAxisB=+Y  BaseAlignAxisB=+Z  RotationSequenceAxes=FollowerAxes  RotationSequence=XYX  RotationSequenceAngles=[0 0 0]  RotationSequenceAnglesUnits=deg  RotationMatrix=[1 0 0; 0 1 0; 0 0 1]
  Solid : sm_lib/Body Elements/Solid  InertiaType=PointMass  Mass=0.00001  MassUnits=kg  CenterOfMass=[0 0 0]  CenterOfMassUnits=m  MomentsOfInertia=[1 1 1]  MomentsOfInertiaUnits=kg*m^2  ProductsOfInertia=[1 1 1]  ProductsOfInertiaUnits=kg*m^2  DensityBased=on  Density=1000  DensityUnits=kg/m^3  DoExposeReferenceFrame=on  SerializedFrames=<Frames/>  GraphicType=FromGeometry  MarkerShape=Sphere  MarkerSize=10  GraphicVisPropType=SimpleVisualProperties  GraphicDiffuseColor=[0.5 0.5 0.5]  GraphicSpecularColor=[0.5 0.5 0.5 1.0]  GraphicAmbientColor=[0.15 0.15 0.15 1.0]  GraphicEmissiveColor=[0.0 0.0 0.0 1.0]  GraphicShininess=75  GraphicOpacity=0  GeometryShape=Brick  RectangleSize=[1 1]  RectangleSizeUnits=m  BrickDimensions=[0.001 0.001 0.001]  BrickDimensionUnits=m  CylinderRadius=1  CylinderRadiusUnits=m  CylinderLength=1  CylinderLengthUnits=m  SphereRadius=1  SphereRadiusUnits=m  EllipsoidRadii=[1 1 1]  EllipsoidRadiiUnits=m  ExtrusionCrossSection=[1 1; -1 1; -1 -1; 1 -1]  ExtrusionCrossSectionUnits=m  ExtrusionLength=1  ExtrusionLengthUnits=m  PolygonNumSides=3  PolygonOuterRadius=1  PolygonOuterRadiusUnits=m  ExtGeomFileType=STEP  ExtGeomFileUnits=m  RevolutionCrossSection=[1 1; 1 -1; 2 -1; 2 1]  RevolutionCrossSectionUnits=m  RevolutionExtent=Full  RevolutionAngle=180  RevolutionAngleUnits=deg
  Robot : PMIOPort  Side=Left
  connections:
  RobotCamera/RConn1 -- Solid/RConn1
  Arrow/RConn1 -- Robot/RConn1 -- RobotCamera/LConn1 -- Base/RConn1

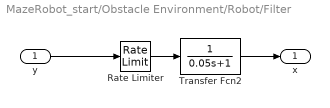
== system MazeRobot_start/Obstacle Environment/Robot/Filter ==
  y : Inport
  Rate Limiter : RateLimiter  RisingSlewLimit=300  FallingSlewLimit=-300  SampleTimeMode=inherited
  Transfer Fcn2 : TransferFcn  Denominator=[0.05 1]
  x : Outport
  wires:
  Rate Limiter/1 -> Transfer Fcn2/1
  Transfer Fcn2/1 -> x/1
  y/1 -> Rate Limiter/1

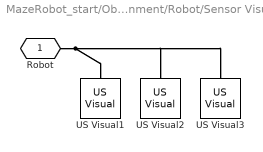
== system MazeRobot_start/Obstacle Environment/Robot/Sensor Visuals ==
  US Visual1 : RP_Simulator_Components/US Visual  size=1  color=[0.5 0.1 0.1]  pose=[0.25 0]  angle=0
  US Visual2 : RP_Simulator_Components/US Visual  size=1  color=[0.5 0.1 0.1]  pose=[0.15 0.15]  angle=90
  US Visual3 : RP_Simulator_Components/US Visual  size=1  color=[0.5 0.1 0.1]  pose=[0.15 -0.15]  angle=-90
  Robot : PMIOPort  Side=Left
  connections:
  US Visual1/LConn1 -- Robot/RConn1 -- US Visual2/LConn1 -- US Visual3/LConn1

== stateflow chart MazeRobot_start/Navigate Maze ==
  state TurnLeft
  state TurnRight
  state MoveForward
  (default) -> MoveForward
  MoveForward -> TurnLeft [order 2]
  MoveForward -> TurnRight [order 1]
  TurnRight -> MoveForward
  TurnLeft -> MoveForward
  data: LeftMotor output; RightMotor output; frontDist input; leftDist input; rightDist input
